simulink model "INPUT"  (R2024b)
settings: configuration reference "STM32H7_Config" (kept outside this file)
settings Model: DataDictionary=Master_Dictionary.sldd  EnableAccessToBaseWorkspace=off  Creator=torni  LastModifiedBy=oxbro
settings ConfigSetRef: SourceName=STM32H7_Config

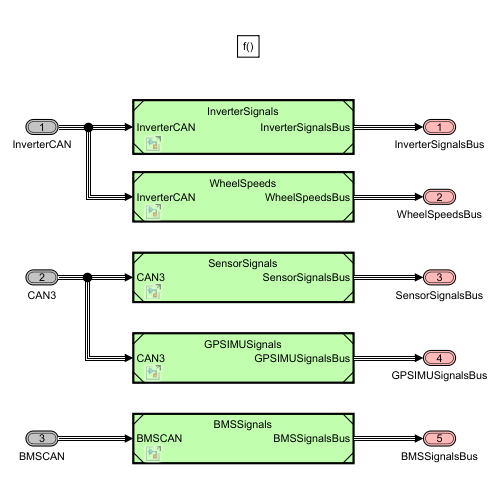
[thumbnail: Simulink's stored preview of the top-level diagram]
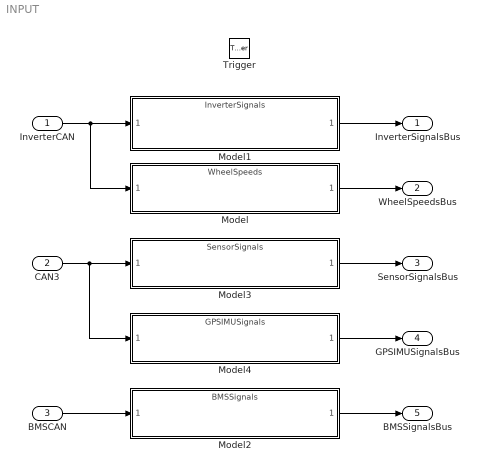
== system INPUT ==
  InverterCAN : Inport  OutDataTypeStr=Bus: CAN1_2Bus
  CAN3 : Inport  Port=2  OutDataTypeStr=Bus: CAN3Bus
  BMSCAN : Inport  Port=3  OutDataTypeStr=Bus: CAN4Bus
  Trigger : TriggerPort  TriggerType=function-call  VariantControl=(inherit)  SampleTime=-1  InitialTriggerSignalState=positive  PortDimensions=1
  Model : ModelReference  ModelNameDialog=WheelSpeeds.slx  SimulationMode=Normal  ModelReferenceVersion=13.6
  Model1 : ModelReference  ModelNameDialog=InverterSignals.slx  SimulationMode=Normal  ModelReferenceVersion=13.10
  Model2 : ModelReference  ModelNameDialog=BMSSignals.slx  SimulationMode=Normal  ModelReferenceVersion=13.7
  Model3 : ModelReference  ModelNameDialog=SensorSignals.slx  SimulationMode=Normal  ModelReferenceVersion=13.6
  Model4 : ModelReference  ModelNameDialog=GPSIMUSignals.slx  SimulationMode=Normal  ModelReferenceVersion=13.7
  InverterSignalsBus : Outport  OutDataTypeStr=Bus: InverterSignalsBus  VectorParamsAs1DForOutWhenUnconnected=off
  WheelSpeedsBus : Outport  Port=2  OutDataTypeStr=Bus: WheelSpeedsBus  VectorParamsAs1DForOutWhenUnconnected=off
  SensorSignalsBus : Outport  Port=3  OutDataTypeStr=Bus: SensorSignalsBus  VectorParamsAs1DForOutWhenUnconnected=off
  GPSIMUSignalsBus : Outport  Port=4  OutDataTypeStr=Bus: GPSIMUSignalsBus  VectorParamsAs1DForOutWhenUnconnected=off
  BMSSignalsBus : Outport  Port=5  OutDataTypeStr=Bus: BMSSignalsBus  VectorParamsAs1DForOutWhenUnconnected=off
  wires:
  Model/1 -> WheelSpeedsBus/1
  Model1/1 -> InverterSignalsBus/1
  CAN3/1 -> Model4/1, Model3/1
  InverterCAN/1 -> Model1/1, Model/1
  Model2/1 -> BMSSignalsBus/1
  BMSCAN/1 -> Model2/1
  Model3/1 -> SensorSignalsBus/1
  Model4/1 -> GPSIMUSignalsBus/1
